simulink model "chapter9_2"  (R2019a)
settings: Solver=ode45  StartTime=0.0  StopTime=20  RelTol=1e-3
settings Model: Creator=ZUNAED  LastModifiedBy=ZUNAED

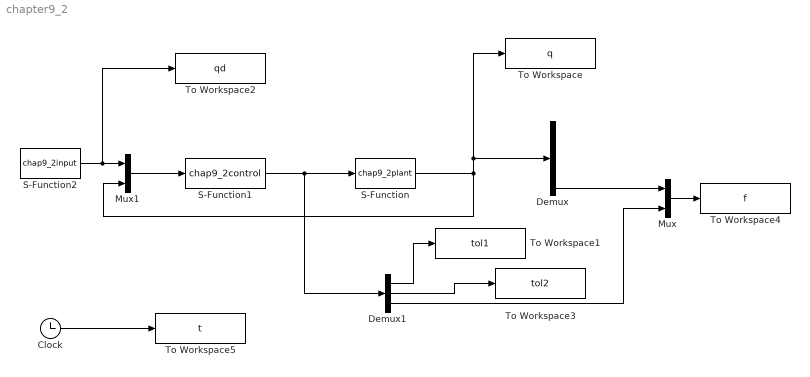
== system chapter9_2 ==
  Clock : Clock
  Demux : Demux  Outputs=5
  Demux1 : Demux  Outputs=3
  Mux : Mux  Inputs=2
  Mux1 : Mux  Inputs=2
  S-Function : S-Function  FunctionName=chap9_2plant  SFunctionDeploymentMode=off  EnableBusSupport=off
  S-Function1 : S-Function  FunctionName=chap9_2control  SFunctionDeploymentMode=off  EnableBusSupport=off
  S-Function2 : S-Function  FunctionName=chap9_2input  SFunctionDeploymentMode=off  EnableBusSupport=off
  To Workspace : ToWorkspace  VariableName=q  SaveFormat=Timeseries  SampleTime=-1
  To Workspace1 : ToWorkspace  VariableName=tol1  SaveFormat=Timeseries  SampleTime=-1
  To Workspace2 : ToWorkspace  VariableName=qd  SaveFormat=Timeseries  SampleTime=-1
  To Workspace3 : ToWorkspace  VariableName=tol2  SaveFormat=Timeseries  SampleTime=-1
  To Workspace4 : ToWorkspace  VariableName=f  SaveFormat=Timeseries  SampleTime=-1
  To Workspace5 : ToWorkspace  VariableName=t  SaveFormat=Timeseries  SampleTime=-1
  wires:
  S-Function2/1 -> To Workspace2/1, Mux1/1
  Mux1/1 -> S-Function1/1
  S-Function1/1 -> Demux1/1, S-Function/1
  S-Function/1 -> To Workspace/1, Demux/1, Mux1/2
  Demux1/3 -> Mux/2
  Clock/1 -> To Workspace5/1
  Demux1/1 -> To Workspace1/1
  Demux1/2 -> To Workspace3/1
  Mux/1 -> To Workspace4/1
  Demux/5 -> Mux/1
